simulink model "LQR"  (R2020a)
settings: Solver=VariableStepAuto  StartTime=0.0  StopTime=200  RelTol=1e-3
undefined symbols (not defined in the file): c_s, K_LQR, ki_LQR, kr
libraries: fl_lib x15, nesl_utility x9, simulink x2
settings Model: Creator=juan  LastModifiedBy=juan

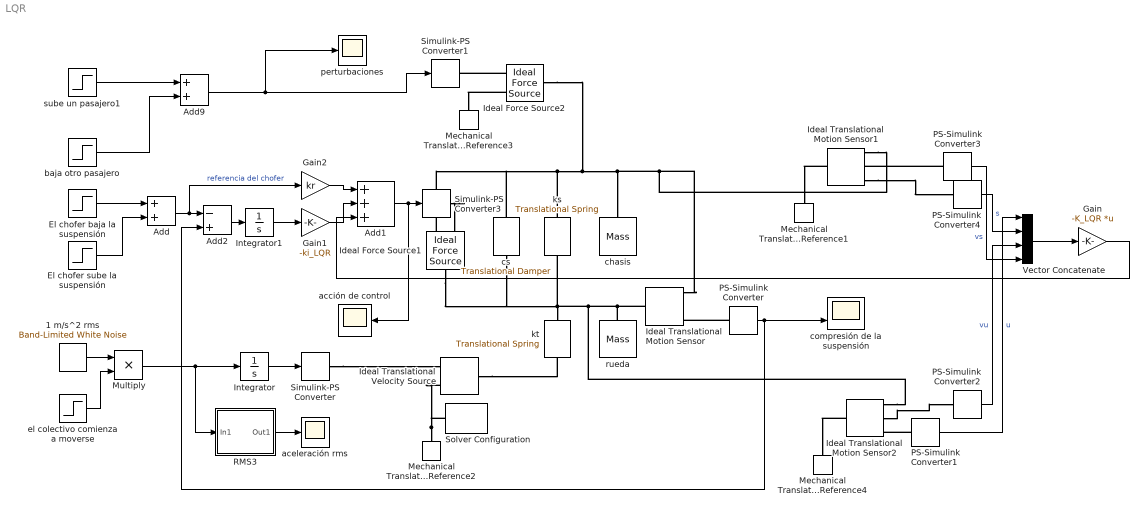
== system LQR ==
  1 m/s^2 rms : simulink/Sources/Band-Limited White Noise  Cov=(1^2)/(1/0.1)  Ts=0.1  seed=[95647]
  Add : Sum
  Add1 : Sum  Inputs=+++
  Add2 : Sum  Inputs=-+
  Add9 : Sum
  El chofer baja la suspensión : Step  Time=10  After=-0.15  SampleTime=0
  El chofer sube la suspensión : Step  Time=30  After=.15  SampleTime=0
  Gain : Gain  Gain=-K_LQR  Multiplication=Matrix(K*u)
  Gain1 : Gain  Gain=-ki_LQR
  Gain2 : Gain  Gain=kr
  Ideal Force Source1 : fl_lib/Mechanical/Mechanical Sources/Ideal Force Source
  Ideal Force Source2 : fl_lib/Mechanical/Mechanical Sources/Ideal Force Source
  Ideal Translational Motion Sensor : fl_lib/Mechanical/Mechanical Sensors/Ideal Translational Motion Sensor  offset=0 m
  Ideal Translational Motion Sensor1 : fl_lib/Mechanical/Mechanical Sensors/Ideal Translational Motion Sensor  offset=0 m
  Ideal Translational Motion Sensor2 : fl_lib/Mechanical/Mechanical Sensors/Ideal Translational Motion Sensor  offset=0 m
  Ideal Translational Velocity Source : fl_lib/Mechanical/Mechanical Sources/Ideal Translational Velocity Source
  Integrator : Integrator
  Integrator1 : Integrator
  Mechanical Translational Reference{1..4} (4 alike) : fl_lib/Mechanical/Translational Elements/Mechanical Translational Reference
  Multiply : Product
  PS-Simulink Converter{,1..4} (5 alike) : nesl_utility/PS-Simulink Converter  PhysicalDomain=network_engine_domain  SubClassName=ps_output  LeftPortType=input  RightPortType=output  PseudoPeriodic=off  Frequencies=[]  Unit=1  AffineConversion=off
  RMS3 : Subsystem
  Simulink-PS Converter : nesl_utility/Simulink-PS Converter  PhysicalDomain=network_engine_domain  SubClassName=ps_input  LeftPortType=input  RightPortType=output  PseudoPeriodic=off  Frequencies=[]  NoiseDistribution=none  NoiseParameters=[]  Unit=1  AffineConversion=off  FilteringAndDerivatives=provide  SimscapeFilterOrder=1  InputFilterTimeConstant=0.001  UdotUserProvided=0
  Simulink-PS Converter1 : nesl_utility/Simulink-PS Converter  PhysicalDomain=network_engine_domain  SubClassName=ps_input  LeftPortType=input  RightPortType=output  PseudoPeriodic=off  Frequencies=[]  NoiseDistribution=none  NoiseParameters=[]  Unit=1  AffineConversion=off  FilteringAndDerivatives=provide  SimscapeFilterOrder=1  InputFilterTimeConstant=0.001  UdotUserProvided=0
  Simulink-PS Converter3 : nesl_utility/Simulink-PS Converter  PhysicalDomain=network_engine_domain  SubClassName=ps_input  LeftPortType=input  RightPortType=output  PseudoPeriodic=off  Frequencies=[]  NoiseDistribution=none  NoiseParameters=[]  Unit=1  AffineConversion=off  FilteringAndDerivatives=provide  SimscapeFilterOrder=1  InputFilterTimeConstant=0.001  UdotUserProvided=0
  Solver Configuration : nesl_utility/Solver Configuration  PhysicalDomain=network_engine_domain  SubClassName=solver  LeftPortType=input  RightPortType=generic  Tones=[]  Harmonics=[]  SimulateNoise=off  Profile=off  UseLocalSampling=off  EnableSwitchedLinearOptims=on  FrequencyDomain=off  UseCCode=off  RelTol=0.001  AbsTol=1e-06  MinStep=1e-09  ToWorkspace=off  RevertToSquareIcSolve=off  NumHomotopyIterations=100  PhasorMode=off  PhasorModeNumHarmonics=1  DoDC=off  ResidualTolerance=1e-09  UseLocalSolver=off  LocalSolverChoice=NE_BACKWARD_EULER_ADVANCER  LocalSolverSampleTime=0.001  DoFixedCost=off  MaxNonlinIter=3  MaxModeIter=2  LinearAlgebra=Sparse  EquationFormulation=NE_TIME_EF  DelaysMemoryBudget=1024  AutomaticFiltering=on  FilteringTimeConstant=0.001  PartitionStorageMethod=AS_NEEDED  PartitionMemoryBudget=1024  PartitionMethod=FAST
  Vector Concatenate : Concatenate  NumInputs=4
  acción de control : Scope
  aceleración rms : Scope
  baja otro pasajero : Step  Time=25  After=-700  SampleTime=0
  chasis : fl_lib/Mechanical/Translational Elements/Mass  mass=m_s kg  v_specify=off  v_priority=High  v=0 m/s  v_nominal_specify=off  v_nominal_unit=m/s  v_nominal_value=1  f_specify=off  f_priority=None  f=0 N  f_nominal_specify=off  f_nominal_unit=N  f_nominal_value=1
  compresión de la suspensión : Scope  NumInputPorts=2
  cs : fl_lib/Mechanical/Translational Elements/Translational Damper  D=c_s N/(m/s)  v_specify=off  v_priority=None  v=0 m/s  v_nominal_specify=off  v_nominal_unit=m/s  v_nominal_value=1  f_specify=off  f_priority=None  f=0 N  f_nominal_specify=off  f_nominal_unit=N  f_nominal_value=1
  el colectivo comienza a moverse : Step  Time=50  SampleTime=0
  ks : fl_lib/Mechanical/Translational Elements/Translational Spring  spr_rate=k_s N/m  v_specify=off  v_priority=None  v=0 m/s  v_nominal_specify=off  v_nominal_unit=m/s  v_nominal_value=1  f_specify=off  f_priority=None  f=0 N  f_nominal_specify=off  f_nominal_unit=N  f_nominal_value=1  x_specify=off  x_priority=High  x=0 m  x_nominal_specify=off  x_nominal_unit=m  x_nominal_value=1
  kt : fl_lib/Mechanical/Translational Elements/Translational Spring  spr_rate=k_t N/m  v_specify=off  v_priority=None  v=0 m/s  v_nominal_specify=off  v_nominal_unit=m/s  v_nominal_value=1  f_specify=off  f_priority=None  f=0 N  f_nominal_specify=off  f_nominal_unit=N  f_nominal_value=1  x_specify=off  x_priority=High  x=0 m  x_nominal_specify=off  x_nominal_unit=m  x_nominal_value=1
  perturbaciones : Scope
  rueda : fl_lib/Mechanical/Translational Elements/Mass  mass=m_u kg  v_specify=off  v_priority=High  v=0 m/s  v_nominal_specify=off  v_nominal_unit=m/s  v_nominal_value=1  f_specify=off  f_priority=None  f=0 N  f_nominal_specify=off  f_nominal_unit=N  f_nominal_value=1
  sube un pasajero1 : Step  Time=20  After=700  SampleTime=0
  wires:
  PS-Simulink Converter1/1 -> Vector Concatenate/1  "u"
  sube un pasajero1/1 -> Add9/1
  Integrator/1 -> Simulink-PS Converter/1
  PS-Simulink Converter/1 -> Add2/2, compresión de la suspensión/2
  Add9/1 -> Simulink-PS Converter1/1, perturbaciones/1
  baja otro pasajero/1 -> Add9/2
  El chofer baja la suspensión/1 -> Add/1
  el colectivo comienza a moverse/1 -> Multiply/2
  PS-Simulink Converter3/1 -> Vector Concatenate/4  "vs"
  PS-Simulink Converter4/1 -> Vector Concatenate/2  "s"
  RMS3/1(Out1) -> aceleración rms/1
  Multiply/1 -> RMS3/1(In1), Integrator/1
  El chofer sube la suspensión/1 -> Add/2
  1 m/s^2 rms/1 -> Multiply/1
  PS-Simulink Converter2/1 -> Vector Concatenate/3  "vu"
  Vector Concatenate/1 -> Gain/1
  Add1/1 -> acción de control/1, Simulink-PS Converter3/1
  Gain/1 -> Add1/3
  Add/1 -> Gain2/1, Add2/1  "referencia del chofer"
  Add2/1 -> Integrator1/1
  Integrator1/1 -> Gain1/1
  Gain1/1 -> Add1/2
  Gain2/1 -> Add1/1
  connections:
  Mechanical Translational Reference2/LConn1 -- Ideal Translational Velocity Source/RConn2 -- Solver Configuration/RConn1
  Ideal Translational Motion Sensor/LConn1 -- kt/RConn1 -- cs/LConn1 -- Ideal Force Source1/LConn1 -- ks/LConn1 -- Ideal Translational Motion Sensor2/RConn1 -- rueda/LConn1
  Ideal Translational Motion Sensor1/RConn1 -- Ideal Translational Motion Sensor/RConn1 -- ks/RConn1 -- Ideal Force Source1/RConn2 -- cs/RConn1 -- Ideal Force Source2/LConn1 -- chasis/LConn1
  Ideal Translational Velocity Source/LConn1 -- kt/LConn1
  Simulink-PS Converter/RConn1 -- Ideal Translational Velocity Source/RConn1
  PS-Simulink Converter3/LConn1 -- Ideal Translational Motion Sensor1/RConn2
  PS-Simulink Converter/LConn1 -- Ideal Translational Motion Sensor/RConn3
  Simulink-PS Converter3/RConn1 -- Ideal Force Source1/RConn1
  Ideal Translational Motion Sensor1/LConn1 -- Mechanical Translational Reference1/LConn1
  PS-Simulink Converter1/LConn1 -- Ideal Translational Motion Sensor2/RConn3
  Ideal Force Source2/RConn1 -- Simulink-PS Converter1/RConn1
  Ideal Translational Motion Sensor1/RConn3 -- PS-Simulink Converter4/LConn1
  Ideal Translational Motion Sensor2/RConn2 -- PS-Simulink Converter2/LConn1
  Ideal Force Source2/RConn2 -- Mechanical Translational Reference3/LConn1
  Ideal Translational Motion Sensor2/LConn1 -- Mechanical Translational Reference4/LConn1

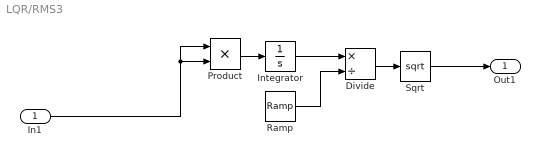
== system LQR/RMS3 ==
  In1 : Inport
  Divide : Product  Inputs=*/
  Integrator : Integrator
  Product : Product
  Ramp : simulink/Sources/Ramp  slope=1  start=0  InitialOutput=0
  Sqrt : Sqrt  SaturateOnIntegerOverflow=on
  Out1 : Outport  VectorParamsAs1DForOutWhenUnconnected=off
  wires:
  Ramp/1 -> Divide/2
  Product/1 -> Integrator/1
  Integrator/1 -> Divide/1
  Sqrt/1 -> Out1/1
  Divide/1 -> Sqrt/1
  In1/1 -> Product/1, Product/2
